simulink library "ECE1718_cnn_original"  (R2022b)
settings: Solver=VariableStepAuto  StartTime=0.0  StopTime=10.0  RelTol=1e-3
libraries: $bdroot x2
(part 1 of 2)
settings Model: Creator=kevin  LastModifiedBy=kevin
settings SFSimCC: SimCustomHeaderCode="#include \"interface-1.h\""  SimUserSources=./cnn_mnist-1.cpp  SimUserIncludeDirs=./../../../../usr/include/c++/11  SimAnalyzeCustomCode=on  CustomCodeGlobalsAsFunctionIO=on  DefaultCustomCodeDeterministicFunctions=All  SimTargetLang=C++
settings RTWCC: RTWUseSimCustomCode=on  CustomHeaderCode="#include \"interface-1.h\""  CustomInclude=./../../../../usr/include/c++/11  CustomSource=./cnn_mnist-1.cpp

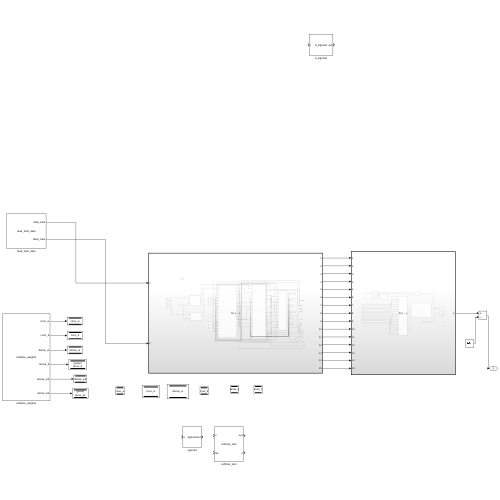
[thumbnail: Simulink's stored preview of the top-level diagram]
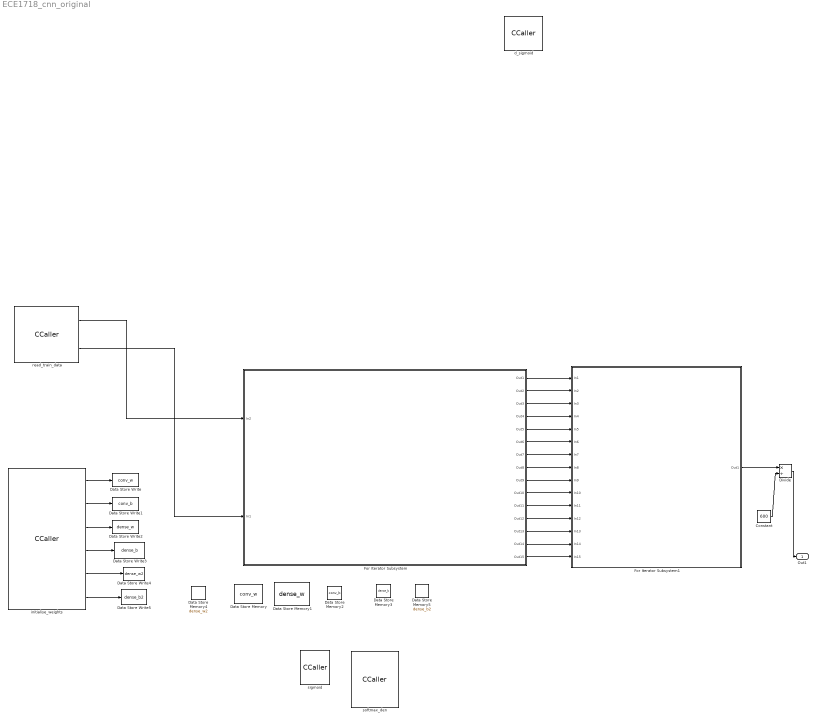
== system ECE1718_cnn_original ==
  Constant : Constant  Value=600
  Data Store Memory : DataStoreMemory  DataStoreName=conv_w  WriteAfterWriteMsg=warning  ShowAdditionalParam=off
  Data Store Memory1 : DataStoreMemory  DataStoreName=dense_w  WriteAfterWriteMsg=warning  ShowAdditionalParam=off
  Data Store Memory2 : DataStoreMemory  DataStoreName=conv_b  WriteAfterWriteMsg=warning  ShowAdditionalParam=off
  Data Store Memory3 : DataStoreMemory  DataStoreName=dense_b  WriteAfterWriteMsg=warning  ShowAdditionalParam=off
  Data Store Memory4 : DataStoreMemory  DataStoreName=dense_w2  WriteAfterWriteMsg=warning  ShowAdditionalParam=off
  Data Store Memory5 : DataStoreMemory  DataStoreName=dense_b2  WriteAfterWriteMsg=warning  ShowAdditionalParam=off
  Data Store Write : DataStoreWrite  DataStoreName=conv_w  IndexOptions=Index vector (dialog)  Indices=1  OutputSizes=1
  Data Store Write1 : DataStoreWrite  DataStoreName=conv_b  IndexOptions=Index vector (dialog)  Indices=1  OutputSizes=1
  Data Store Write2 : DataStoreWrite  DataStoreName=dense_w  IndexOptions=Index vector (dialog)  Indices=1  OutputSizes=1
  Data Store Write3 : DataStoreWrite  DataStoreName=dense_b  IndexOptions=Index vector (dialog)  Indices=1  OutputSizes=1
  Data Store Write4 : DataStoreWrite  DataStoreName=dense_w2  IndexOptions=Index vector (dialog)  Indices=1  OutputSizes=1
  Data Store Write5 : DataStoreWrite  DataStoreName=dense_b2  IndexOptions=Index vector (dialog)  Indices=1  OutputSizes=1
  Divide : Product  Inputs=*/
  For Iterator Subsystem : Subsystem  TreatAsAtomicUnit=on
  For Iterator Subsystem1 : Subsystem  TreatAsAtomicUnit=on
  d_sigmoid : CCaller  FunctionName=d_sigmoid  PortSpecificationStruct="%)30     .    N ,   8    (     @         %    \"     (    !     0         %  0 \"0    $    _    07)G3F%M90  4&]R=$YA;64 4V-O<&4     26YD97@     5'EP90      4VEZ90      27-';&]B86P   X    P    !@    @    $          4    (     0    ,    !         !   P!O=70 #@   #     &    \"     0         !0    @    !     P    $         $  # &]U=  .    .     8    (    !          %    \"     $    &     0         0    !@   $]U='!U=   #@   #@    &    \"     8         !0    @    !     0    $         \"0    @               X    X    !@    @    $          4    (     0    8    !         !     &    9&]U8FQE   .    ,     8    (    !          %    \"     $    !     0         0  $ ,0    X    P    !@    @    ) @        4    (     0    $    !          (  0      #@   #     &    \"     0         !0    @    !     0    $         $  ! '@    .    ,     8    (    !          %    \"     $    !     0         0  $ >     X    X    !@    @    $          4    (     0    4    !         !     %    26YP=70    .    .     8    (    !@         %    \"     $    !     0         )    \"               #@   #@    &    \"     0         !0    @    !    !@    $         $     8   !D;W5B;&4   X    P    !@    @    $          4    (     0    $    !         !   0 Q    #@   #     &    \"     D\"        !0    @    !     0    $          @ !"
  initialise_weights : CCaller  FunctionName=initialise_weights  PortSpecificationStruct="%)30     .    H H   8    (     @         %    \"     8    !     0         %  0 \"0    $    _    07)G3F%M90  4&]R=$YA;64 4V-O<&4     26YD97@     5'EP90      4VEZ90      27-';&]B86P   X    X    !@    @    $          4    (     0    8    !         !     &    8V]N=E]W   .    .     8    (    !          %    \"     $    &     0         0    !@   &-O;G9?=P  #@   #@    &    \"     0         !0    @    !   ...(+3280 chars)"
  read_train_data : CCaller  FunctionName=read_train_data  PortSpecificationStruct="%)30     .    & 0   8    (     @         %    \"     (    !     0         %  0 \"0    $    _    07)G3F%M90  4&]R=$YA;64 4V-O<&4     26YD97@     5'EP90      4VEZ90      27-';&]B86P   X   !     !@    @    $          4    (     0    H    !         !     *    9&%T85]T<F%I;@        X   !     !@    @    $          4    (     0    H    !         !     *    9&%T85]T<F%I;@        X    X    !@    @    $          4    (     0    8    !         !     &    3W5T<'5T   .    .     8    (    !@         %    \"     $    !     0         )    \"               #@   $     &    \"     0         !0    @    !    $     $         $    !    !F:7AD=\"@P+#@L,EXP+# I#@   #@    &    \"     0         !0    @    !    \"     $         $     @    T-S T,# P, X    P    !@    @    ) @        4    (     0    $    !          (  0      #@   $     &    \"     0         !0    @    !    \"P    $         $     L   !L86)E;%]T<F%I;@      #@   $     &    \"     0         !0    @    !    \"P    $         $     L   !L86)E;%]T<F%I;@      #@   #@    &    \"     0         !0    @    !    !@    $         $     8   !/=71P=70   X    X    !@    @    &          4    (     0    $    !          D    (            \\#\\.    0     8    (    !          %    \"     $    0     0         0    $    &9I>&1T*# L.\"PR7C L,\"D.    .     8    (    !          %    \"     $    %     0         0    !0   #8P,# P    #@   #     &    \"     D\"        !0    @    !     0    $          @ !"
  sigmoid : CCaller  FunctionName=sigmoid  PortSpecificationStruct="%)30     .    N ,   8    (     @         %    \"     (    !     0         %  0 \"0    $    _    07)G3F%M90  4&]R=$YA;64 4V-O<&4     26YD97@     5'EP90      4VEZ90      27-';&]B86P   X    P    !@    @    $          4    (     0    ,    !         !   P!O=70 #@   #     &    \"     0         !0    @    !     P    $         $  # &]U=  .    .     8    (    !          %    \"     $    &     0         0    !@   $]U='!U=   #@   #@    &    \"     8         !0    @    !     0    $         \"0    @               X    X    !@    @    $          4    (     0    8    !         !     &    9&]U8FQE   .    ,     8    (    !          %    \"     $    !     0         0  $ ,0    X    P    !@    @    ) @        4    (     0    $    !          (  0      #@   #     &    \"     0         !0    @    !     0    $         $  ! '@    .    ,     8    (    !          %    \"     $    !     0         0  $ >     X    X    !@    @    $          4    (     0    4    !         !     %    26YP=70    .    .     8    (    !@         %    \"     $    !     0         )    \"               #@   #@    &    \"     0         !0    @    !    !@    $         $     8   !D;W5B;&4   X    P    !@    @    $          4    (     0    $    !         !   0 Q    #@   #     &    \"     D\"        !0    @    !     0    $          @ !"
  softmax_den : CCaller  FunctionName=softmax_den  PortSpecificationStruct="%)30     .    8 4   8    (     @         %    \"     ,    !     0         %  0 \"0    $    _    07)G3F%M90  4&]R=$YA;64 4V-O<&4     26YD97@     5'EP90      4VEZ90      27-';&]B86P   X    P    !@    @    $          4    (     0    ,    !         !   P!O=70 #@   #     &    \"     0         !0    @    !     P    $         $  # &]U=  .    .     8    (    !          %    \"     $    &     0         0    !@   $]U='!U=   #@   #@    &    \"     8         !0    @    !     0    $         \"0    @               X    X    !@    @    $          4    (     0    8    !         !     &    9&]U8FQE   .    ,     8    (    !          %    \"     $    !     0         0  $ ,0    X    P    !@    @    ) @        4    (     0    $    !          (  0      #@   #     &    \"     0         !0    @    !     0    $         $  ! '@    .    ,     8    (    !          %    \"     $    !     0         0  $ >     X   !     !@    @    $          4    (     0    L    !         !     +    26YP=71/=71P=70       X    X    !@    @    &          4    (     0    $    !          D    (               .    .     8    (    !          %    \"     $    &     0         0    !@   &1O=6)L90  #@   #     &    \"     0         !0    @    !     @    $         $  \" \"TQ   .    ,     8    (    \"0(        %    \"     $    !     0         \"  $       X    P    !@    @    $          4    (     0    ,    !         !   P!L96X #@   #     &    \"     0         !0    @    !     P    $         $  # &QE;@ .    .     8    (    !          %    \"     $    %     0         0    !0   $EN<'5T    #@   #@    &    \"     8         !0    @    !     0    $         \"0    @           #P/PX    X    !@    @    $          4    (     0    4    !         !     %    :6YT,S(    .    ,     8    (    !          %    \"     $    !     0         0  $ ,0    X    P    !@    @    ) @        4    (     0    $    !          (  0"
  Out1 : Outport
  wires:
  read_train_data/1 -> For Iterator Subsystem/1(In2)
  read_train_data/2 -> For Iterator Subsystem/2(In1)
  initialise_weights/1 -> Data Store Write/1
  initialise_weights/2 -> Data Store Write1/1
  initialise_weights/3 -> Data Store Write2/1
  initialise_weights/4 -> Data Store Write3/1
  initialise_weights/5 -> Data Store Write4/1
  initialise_weights/6 -> Data Store Write5/1
  For Iterator Subsystem/1(Out1) -> For Iterator Subsystem1/1(In1)
  For Iterator Subsystem/2(Out2) -> For Iterator Subsystem1/2(In2)
  For Iterator Subsystem/3(Out3) -> For Iterator Subsystem1/3(In3)
  For Iterator Subsystem/4(Out4) -> For Iterator Subsystem1/4(In4)
  For Iterator Subsystem/5(Out5) -> For Iterator Subsystem1/5(In5)
  For Iterator Subsystem/6(Out6) -> For Iterator Subsystem1/6(In6)
  For Iterator Subsystem/7(Out7) -> For Iterator Subsystem1/7(In7)
  For Iterator Subsystem/8(Out8) -> For Iterator Subsystem1/8(In8)
  For Iterator Subsystem/9(Out9) -> For Iterator Subsystem1/9(In9)
  For Iterator Subsystem/10(Out10) -> For Iterator Subsystem1/10(In10)
  For Iterator Subsystem/11(Out11) -> For Iterator Subsystem1/11(In11)
  For Iterator Subsystem/12(Out12) -> For Iterator Subsystem1/12(In12)
  For Iterator Subsystem/13(Out13) -> For Iterator Subsystem1/13(In13)
  For Iterator Subsystem/14(Out14) -> For Iterator Subsystem1/14(In14)
  For Iterator Subsystem/15(Out15) -> For Iterator Subsystem1/15(In15)
  For Iterator Subsystem1/1(Out1) -> Divide/1
  Constant/1 -> Divide/2
  Divide/1 -> Out1/1

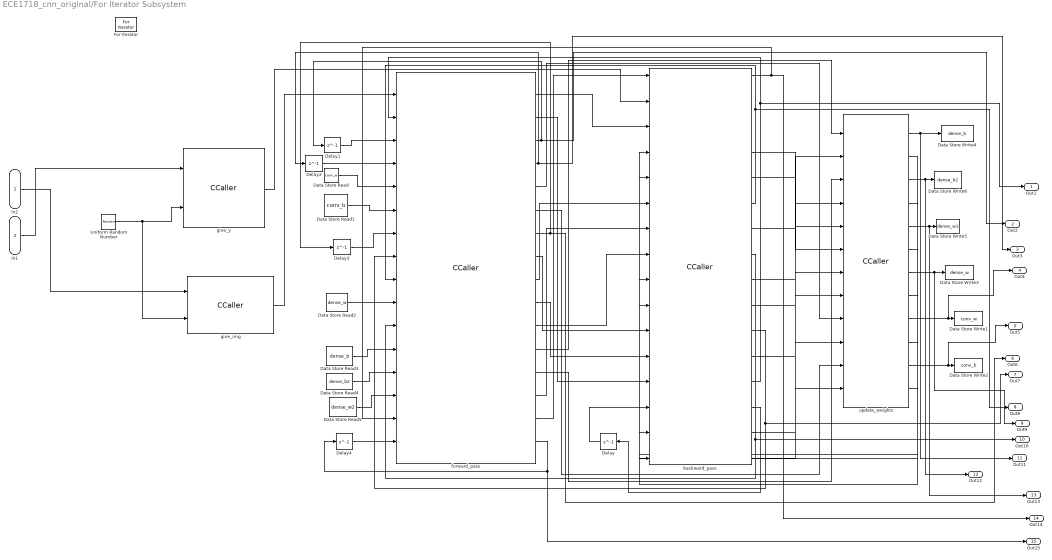
== system ECE1718_cnn_original/For Iterator Subsystem ==
  In2 : Inport  OutDataTypeStr=double  PortDimensions=47040000
  In1 : Inport  Port=2  PortDimensions=60000
  Data Store Read : DataStoreRead  DataStoreName=conv_w  IndexOptions=Index vector (dialog)  Indices=1  OutputSizes=1
  Data Store Read1 : DataStoreRead  DataStoreName=conv_b  IndexOptions=Index vector (dialog)  Indices=1  OutputSizes=1
  Data Store Read2 : DataStoreRead  DataStoreName=dense_w  IndexOptions=Index vector (dialog)  Indices=1  OutputSizes=1
  Data Store Read3 : DataStoreRead  DataStoreName=dense_b  IndexOptions=Index vector (dialog)  Indices=1  OutputSizes=1
  Data Store Read4 : DataStoreRead  DataStoreName=dense_b2  IndexOptions=Index vector (dialog)  Indices=1  OutputSizes=1
  Data Store Read5 : DataStoreRead  DataStoreName=dense_w2  IndexOptions=Index vector (dialog)  Indices=1  OutputSizes=1
  Data Store Write1 : DataStoreWrite  DataStoreName=conv_w  IndexOptions=Index vector (dialog)  Indices=1  OutputSizes=1
  Data Store Write2 : DataStoreWrite  DataStoreName=conv_b  IndexOptions=Index vector (dialog)  Indices=1  OutputSizes=1
  Data Store Write3 : DataStoreWrite  DataStoreName=dense_w  IndexOptions=Index vector (dialog)  Indices=1  OutputSizes=1
  Data Store Write4 : DataStoreWrite  DataStoreName=dense_b  IndexOptions=Index vector (dialog)  Indices=1  OutputSizes=1
  Data Store Write5 : DataStoreWrite  DataStoreName=dense_w2  IndexOptions=Index vector (dialog)  Indices=1  OutputSizes=1
  Data Store Write6 : DataStoreWrite  DataStoreName=dense_b2  IndexOptions=Index vector (dialog)  Indices=1  OutputSizes=1
  Delay{,1..4} (5 alike) : Delay  DelayLength=1  InitialCondition=0
  For Iterator : ForIterator  IterationLimit=500
  Uniform Random Number : UniformRandomNumber  Minimum=0  Maximum=60000
  backward_pass : CCaller  FunctionName=backward_pass  PortSpecificationStruct="%)30     .    T!L   8    (     @         %    \"    !     !     0         %  0 \"0    $    _    07)G3F%M90  4&]R=$YA;64 4V-O<&4     26YD97@     5'EP90      4VEZ90      27-';&]B86P   X    X    !@    @    $          4    (     0    4    !         !     %    >5]H870    .    .     8    (    !          %    \"     $    %     0         0    !0   'E?:&%T    #@   $     &    \"     0         !0    @    !   ...(+9242 chars)"
  forward_pass : CCaller  FunctionName=forward_pass  PortSpecificationStruct="%)30     .    <!P   8    (     @         %    \"    !     !     0         %  0 \"0    $    _    07)G3F%M90  4&]R=$YA;64 4V-O<&4     26YD97@     5'EP90      4VEZ90      27-';&]B86P   X    P    !@    @    $          4    (     0    ,    !         !   P!I;6< #@   #     &    \"     0         !0    @    !     P    $         $  # &EM9P .    0     8    (    !          %    \"     $    +     0         0   ...(+9462 chars)"
  give_img : CCaller  FunctionName=give_img  PortSpecificationStruct="%)30     .    6 4   8    (     @         %    \"     ,    !     0         %  0 \"0    $    _    07)G3F%M90  4&]R=$YA;64 4V-O<&4     26YD97@     5'EP90      4VEZ90      27-';&]B86P   X    P    !@    @    $          4    (     0    ,    !         !   P!V96, #@   #     &    \"     0         !0    @    !     P    $         $  # '9E8P .    .     8    (    !          %    \"     $    %     0         0    !0   $EN<'5T    #@   #@    &    \"     8         !0    @    !     0    $         \"0    @               X    X    !@    @    $          4    (     0    4    !         !     %    =6EN=#@    .    ,     8    (    !          %    \"     $    \"     0         0  ( +3$   X    P    !@    @    ) @        4    (     0    $    !          (  0      #@   #     &    \"     0         !0    @    !     P    $         $  # &EM9P .    ,     8    (    !          %    \"     $    #     0         0  , :6UG  X    X    !@    @    $          4    (     0    8    !         !     &    3W5T<'5T   .    .     8    (    !@         %    \"     $    !     0         )    \"               #@   #@    &    \"     0         !0    @    !    !0    $         $     4   !U:6YT.     X    P    !@    @    $          4    (     0    0    !         !  !  Q,3(P#@   #     &    \"     D\"        !0    @    !     0    $          @ !       .    ,     8    (    !          %    \"     $    #     0         0  , ;G5M  X    P    !@    @    $          4    (     0    ,    !         !   P!N=6T #@   #@    &    \"     0         !0    @    !    !0    $         $     4   !);G!U=     X    X    !@    @    &          4    (     0    $    !          D    (            \\#\\.    .     8    (    !          %    \"     $    %     0         0    !0   &EN=#,R    #@   #     &    \"     0         !0    @    !     0    $         $  ! #$    .    ,     8    (    \"0(        %    \"     $    !     0         \"  $"
  give_y : CCaller  FunctionName=give_y  PortSpecificationStruct="%)30     .    : 4   8    (     @         %    \"     ,    !     0         %  0 \"0    $    _    07)G3F%M90  4&]R=$YA;64 4V-O<&4     26YD97@     5'EP90      4VEZ90      27-';&]B86P   X    P    !@    @    $          4    (     0    $    !         !   0!Y    #@   #     &    \"     0         !0    @    !     0    $         $  ! 'D    .    .     8    (    !          %    \"     $    %     0         0    !0   $EN<'5T    #@   #@    &    \"     8         !0    @    !     0    $         \"0    @               X    X    !@    @    $          4    (     0    4    !         !     %    =6EN=#@    .    ,     8    (    !          %    \"     $    \"     0         0  ( +3$   X    P    !@    @    ) @        4    (     0    $    !          (  0      #@   #@    &    \"     0         !0    @    !    \"     $         $     @   !V96-T;W)?>0X    X    !@    @    $          4    (     0    @    !         !     (    =F5C=&]R7WD.    .     8    (    !          %    \"     $    &     0         0    !@   $]U='!U=   #@   #@    &    \"     8         !0    @    !     0    $         \"0    @               X    X    !@    @    $          4    (     0    4    !         !     %    :6YT,S(    .    ,     8    (    !          %    \"     $    \"     0         0  ( ,3    X    P    !@    @    ) @        4    (     0    $    !          (  0      #@   #     &    \"     0         !0    @    !     P    $         $  # &YU;0 .    ,     8    (    !          %    \"     $    #     0         0  , ;G5M  X    X    !@    @    $          4    (     0    4    !         !     %    26YP=70    .    .     8    (    !@         %    \"     $    !     0         )    \"            / _#@   #@    &    \"     0         !0    @    !    !0    $         $     4   !I;G0S,@    X    P    !@    @    $          4    (     0    $    !         !   0 Q    #@   #     &    \"     D\"        !0    @    !     0    $          @ !"
  update_weights : CCaller  FunctionName=update_weights  PortSpecificationStruct="%)30     .    V!0   8    (     @         %    \"     P    !     0         %  0 \"0    $    _    07)G3F%M90  4&]R=$YA;64 4V-O<&4     26YD97@     5'EP90      4VEZ90      27-';&]B86P   X    X    !@    @    $          4    (     0    <    !         !     '    9&5N<V5?8@ .    .     8    (    !          %    \"     $    '     0         0    !P   &1E;G-E7V( #@   $     &    \"     0         !0    @    !   ...(+6831 chars)"
  Out1 : Outport
  Out2 : Outport  Port=2
  Out3 : Outport  Port=3
  Out4 : Outport  Port=4
  Out5 : Outport  Port=5
  Out6 : Outport  Port=6
  Out7 : Outport  Port=7
  Out8 : Outport  Port=8
  Out9 : Outport  Port=9
  Out10 : Outport  Port=10
  Out11 : Outport  Port=11
  Out12 : Outport  Port=12
  Out13 : Outport  Port=13
  Out14 : Outport  Port=14
  Out15 : Outport  Port=15
  wires:
  backward_pass/12 -> update_weights/7
  forward_pass/8 -> backward_pass/11
  backward_pass/16 -> update_weights/12
  forward_pass/2 -> backward_pass/13
  forward_pass/13 -> update_weights/3
  give_img/1 -> forward_pass/1
  forward_pass/1 -> backward_pass/3
  In2/1 -> give_img/1
  forward_pass/11 -> backward_pass/8
  backward_pass/5 -> update_weights/6
  forward_pass/12 -> update_weights/1
  give_y/1 -> backward_pass/2
  forward_pass/9 -> backward_pass/6
  backward_pass/15 -> update_weights/10
  forward_pass/14 -> backward_pass/7
  backward_pass/4 -> update_weights/4
  backward_pass/9 -> update_weights/2
  forward_pass/15 -> backward_pass/1
  backward_pass/10 -> update_weights/8
  In1/1 -> give_y/1
  forward_pass/10 -> backward_pass/12
  backward_pass/7 -> update_weights/5
  backward_pass/13 -> forward_pass/2, Out1/1
  forward_pass/3 -> Delay1/1, Out2/1
  forward_pass/4 -> Out3/1, Delay2/1
  forward_pass/7 -> Delay3/1, Out6/1
  backward_pass/11 -> Out7/1, forward_pass/8
  backward_pass/6 -> Out8/1, forward_pass/9
  backward_pass/8 -> forward_pass/11, Out10/1
  backward_pass/1 -> Out14/1, forward_pass/15
  forward_pass/16 -> Delay4/1, Out15/1
  forward_pass/6 -> update_weights/11
  forward_pass/5 -> update_weights/9
  update_weights/4 -> backward_pass/4
  update_weights/6 -> backward_pass/5
  update_weights/2 -> backward_pass/9
  update_weights/8 -> backward_pass/10
  update_weights/12 -> backward_pass/16
  update_weights/10 -> backward_pass/15
  update_weights/9 -> Out4/1, Data Store Write1/1
  update_weights/11 -> Out5/1, Data Store Write2/1
  update_weights/7 -> Out9/1, Data Store Write3/1
  update_weights/5 -> Out13/1, Data Store Write5/1
  update_weights/1 -> Out11/1, Data Store Write4/1
  update_weights/3 -> Out12/1, Data Store Write6/1
  Data Store Read/1 -> forward_pass/5
  Data Store Read1/1 -> forward_pass/6
  Data Store Read2/1 -> forward_pass/10
  Data Store Read3/1 -> forward_pass/12
  Data Store Read4/1 -> forward_pass/13
  Data Store Read5/1 -> forward_pass/14
  Uniform Random Number/1 -> give_y/2, give_img/2
  backward_pass/14 -> Delay/1
  Delay/1 -> backward_pass/14
  Delay1/1 -> forward_pass/3
  Delay2/1 -> forward_pass/4
  Delay3/1 -> forward_pass/7
  Delay4/1 -> forward_pass/16
